simulink model "hopper_6dof_CascadeV2"  (R2025a)
settings: Solver=VariableStepAuto  StartTime=0.0  StopTime=20  RelTol=1e-3
values from neighbouring files (symbols this model uses):
  dcg_dMfu_table = [-0.00694531817472 -0.00694178681649 -0.00693828089331 -0.00693480026996 -0.00693134481199 -0.00692791438575 -0.00692450885835 -0.00692112809769 -0.00691777197246 -0.00691444035208 -0.00691113310675 -0.00690785010743 ... (10000 elements, 100x100)]    [cg_I_LUT.mat]    (also in cg_moi_table_generation.m = zeros(length(ox_masses), length(fu_masses)))
  dcg_dMox_table = [-0.00694531817472 0.00355111679481 0.00356856249576 0.00358595402521 0.00360329160721 0.00362057546465 0.00363780581927 0.00365498289166 0.0036721069013 0.00368917806651 0.00370619660452 0.00372316273141 ... (10000 elements, 100x100)]    [cg_I_LUT.mat]    (also in cg_moi_table_generation.m = zeros(length(ox_masses), length(fu_masses)))
  dI_dMfu_table = [0.00582660125 0.00582660125 0.00582660125 0.00582660125 0.00582660125 0.00582660125 0.00582660125 0.00582660125 0.00582660125 0.00582660125 0.00582660125 0.00582660125 ... (90000 elements, 100x100x9)]    [cg_I_LUT.mat]    (also in cg_moi_table_generation.m = zeros(length(ox_masses), length(fu_masses), 9))
  dI_dMox_table = [0.00582660125 0.00582660125 0.00582660125 0.00582660125 0.00582660125 0.00582660125 0.00582660125 0.00582660125 0.00582660125 0.00582660125 0.00582660125 0.00582660125 ... (90000 elements, 100x100x9)]    [cg_I_LUT.mat]    (also in cg_moi_table_generation.m = zeros(length(ox_masses), length(fu_masses), 9))
  engine_cg = IN.engine_cg    [cg_moi_table_generation.m]    (also in cg_moi_test.m = 0.3556)
  fu_masses = [0 0.131313131313 0.262626262626 0.393939393939 0.525252525253 0.656565656566 0.787878787879 0.919191919192 1.05050505051 1.18181818182 1.31313131313 1.44444444444 ... (100 elements, 1x100)]    [cg_I_LUT.mat]    (also in cg_moi_table_generation.m = linspace(0,IN.propulsion.fuel_mass,100))
  ox_masses = [0 0.161616161616 0.323232323232 0.484848484848 0.646464646465 0.808080808081 0.969696969697 1.13131313131 1.29292929293 1.45454545455 1.61616161616 1.77777777778 ... (100 elements, 1x100)]    [cg_I_LUT.mat]    (also in cg_moi_table_generation.m = linspace(0,IN.propulsion.oxidizer_mass,100))
undefined symbols (not defined in the file or in its folder): bp, cg_init, IN, MoI_init, OUT, r_leg_1, r_leg_2, r_leg_3, r_leg_4, TANKS, tbl1, tbl2
libraries: matrix_library x18, slpidlib x13, dspindex x2, aerolibanim x1, SignalEditorBlockLib x1, aerolibutil x1
(part 1 of 3)
settings Model: Creator=asing  LastModifiedBy=Espin
settings DebuggingCC: SignalInfNanChecking=warning

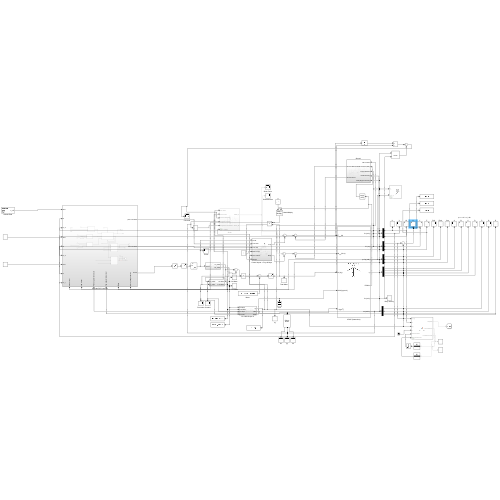
[thumbnail: Simulink's stored preview of the top-level diagram]
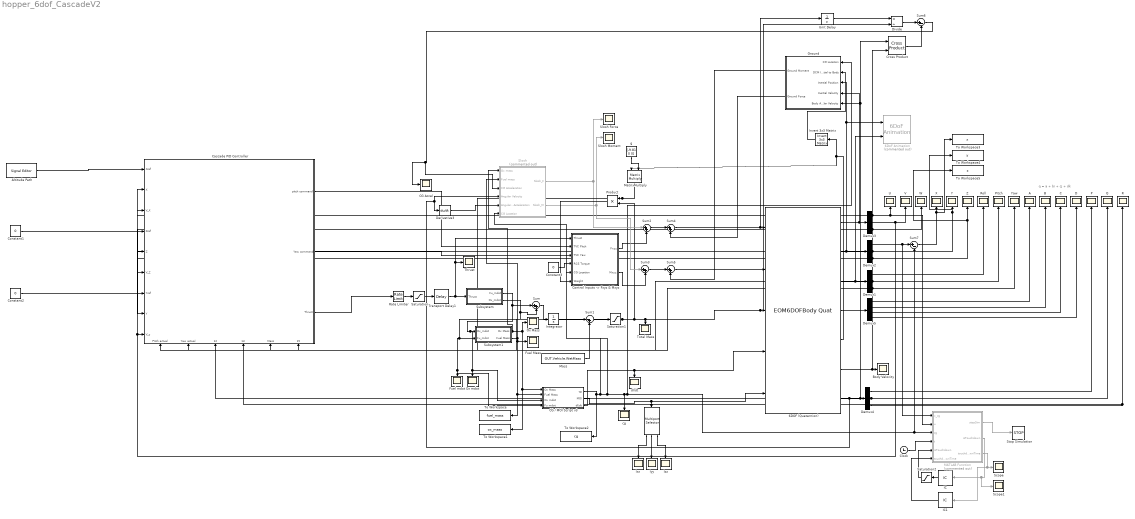
== system hopper_6dof_CascadeV2 ==
  note: q = a + bi + cj + dk
  " " : dspindex/Multiport Selector  rowsOrCols=Rows  idxCellArray={1,2,3}  idxErrMode=Clip Index
      settings: LibrarySourceBlock=|
      | dsphdlsupportsigmgmt/Multiport
      | Selector
  6DOF (Quaternion) : EOM6DOFBodyQuat  mtype=Custom Variable  xme_0=[cg_init 0 0]
  6DoF Animation : aerolibanim/6DoF Animation  Commented=on  u1=[0 4000 -2000 2000 -5000 -3000]  u2=0.1  u3=1.0  u4=[4000 0 -5000]  u5=Fly alongside  u6=[2000 500 -3150]  u7=10  u8=on
  A : Scope
      settings: ActiveDisplayYMinimum=0.99999999995691624  ActiveDisplayYMaximum=1.0000000000047871  DataLoggingVariableName=ScopeData12
  Altitude Path : SignalEditorBlockLib/Signal Editor  FileName=trajectory2.mat  ActiveScenario=scenario  ActiveSignal=z_ref  IsBus=off  OutputBusObjectStr=Bus: BusObject  SampleTime=0  ZeroCross=off  OutputAfterFinalValue=Setting to zero  Unit=inherit  PreserveSignalName=on  ApplySigPropsToAllScenarios=on  ApplySigPropsToAllSignals=off  SignalPropertySource=Dialog parameters
  B : Scope
      settings: ActiveDisplayYMinimum=-1  ActiveDisplayYMaximum=1  DataLoggingVariableName=ScopeData13
  Body Velocity : Scope
      settings: ActiveDisplayYMinimum=-2.8946574443603503  ActiveDisplayYMaximum=19.391983148189578  DataLoggingVariableName=ScopeData29
  C : Scope
      settings: DataLoggingVariableName=ScopeData14
  CG / MOI Script v3 : Subsystem
  CG Accel : Scope
      settings: ActiveDisplayYMinimum=-11.150910258610358  ActiveDisplayYMaximum=2.247247756596932  DataLoggingVariableName=ScopeData33
  Cascade PID Controller : Subsystem
      settings: PortSchema="{\"entries\":[{\"content\":{\"sides\":[{\"content\":{\"connectorIds\":[\"In1\",\"In2\",\"In3\",\"In4\",\"In5\",\"In6\",\"In7\",\"In8\",\"In9\"]},\"type\":\"ConnectorPlacement.EquallySpacedRectSide\",\"uuid\":\"c783e0c4-78fc-4a76-b0b3-9a0d7ec37fa3\"},{\"content\":{\"connectorIds\":[\"Out1\",\"Out2\",\"Out3\"],\"side\":\"RIGHT\"},\"type\":\"ConnectorPlacement.EquallySpacedRectSide\",\"uuid\":\"c1fbc6cd-e8e0-44a7-b5c2-c47c52a42ebb\"},{\"content\":{\"side\":\"TOP\"},\"type\":\"ConnectorPlacement.EquallySpacedRectSide\",\"uuid\":\"09ce9669-ca2f-4231-9dc2-e7ff305f4669\"},{\"content\":{\"connectorIds\":[\"In10\",\"In11\",\"In12\",\"In13\",\"In14\",\"In15\"],\"side\":\"BOTTOM\"},\"type\":\"ConnectorPlacement.EquallySpacedRectSide\",\"uuid\":\"414a52fd-de97-45d1-8e92-1dab180b62e1\"}]},\"type\":\"ConnectorPlacement.EquallySpacedConnector\",\"uuid\":\"cfeff8df-d4aa-41cc-804b-2026e1f59ecf\"}],\"packageUris\":[\"http://schema.mathworks.com/mf0/Connector/R2020b\"],\"version\":\"1.0\"}"
  Clock : Clock
  Constant1 : Constant  Value=0
  Constant2 : Constant  Value=0
  Constant3 : Constant  Value=0
  "Control Inputs -> Fxyz & Mxyz" : Subsystem
  Cross Product : matrix_library/Cross Product
  D : Scope
      settings: DataLoggingVariableName=ScopeData15
  Demux{1..4} (4 alike) : Demux  Outputs=3
  Demux5 : Demux
  Derivative3 : Derivative  CoefficientInTFapproximation=3
  Divide : Product  Inputs=*/
  Fuel Mass : Scope
      settings: ActiveDisplayYMinimum=-1  ActiveDisplayYMaximum=1  DataLoggingVariableName=ScopeData18
  Fuel mdot : Scope
      settings: DataLoggingVariableName=ScopeData20
  "Ground " : Subsystem
  IC : InitialCondition  Value=0
  IC1 : InitialCondition  Value=0
  Integrator : Integrator
  Invert 3x3 Matrix : aerolibutil/Invert  3x3 Matrix
  Ixx : Scope
      settings: ActiveDisplayYMinimum=-0.12644047609192863  ActiveDisplayYMaximum=1.1379642848273579  DataLoggingVariableName=ScopeData21
  Iyy : Scope
      settings: ActiveDisplayYMinimum=-1  ActiveDisplayYMaximum=1  DataLoggingVariableName=ScopeData26
  Izz : Scope
      settings: ActiveDisplayYMinimum=-5.2001669347022288  ActiveDisplayYMaximum=46.801502412320069  DataLoggingVariableName=ScopeData27
  MATLAB Function : MATLAB Function  Commented=on  TreatAsAtomicUnit=on
  Mass : Constant  Value=OUT.Vehicle.WetMass
  MatrixMultiply : Product  Multiplication=Matrix(*)
  Ox Mass : Scope
      settings: ActiveDisplayYMinimum=-1  ActiveDisplayYMaximum=1  DataLoggingVariableName=ScopeData17
  Ox mdot : Scope
      settings: ActiveDisplayYMinimum=-1  ActiveDisplayYMaximum=1  DataLoggingVariableName=ScopeData19
  P : Scope
      settings: ActiveDisplayYMinimum=-1  ActiveDisplayYMaximum=1  DataLoggingVariableName=ScopeData9
  Pitch : Scope
      settings: ActiveDisplayYMinimum=-0.27527761186972155  ActiveDisplayYMaximum=0.20077796412190005  DataLoggingVariableName=ScopeData4
  Product : Product
  Q : Scope
      settings: ActiveDisplayYMinimum=-1  ActiveDisplayYMaximum=1  DataLoggingVariableName=ScopeData10
  R : Scope
      settings: ActiveDisplayYMinimum=-1  ActiveDisplayYMaximum=1  DataLoggingVariableName=ScopeData11
  Rate Limiter : RateLimiter  RisingSlewLimit=IN.throttle_valve.rate_limit  FallingSlewLimit=-IN.throttle_valve.rate_limit  SampleTimeMode=inherited
  Roll : Scope
      settings: ActiveDisplayYMinimum=-3.8311926038814774  ActiveDisplayYMaximum=3.879867078950717  DataLoggingVariableName=ScopeData3
  Saturation : Saturate  UpperLimit=IN.propulsion.nominal_thrust * IN.propulsion.throttle_range(2)  LowerLimit=IN.propulsion.nominal_thrust * IN.propulsion.throttle_range(1)
  Saturation1 : Saturate  UpperLimit=OUT.Vehicle.WetMass  LowerLimit=OUT.Vehicle.DryMass
  Saturation2 : Saturate  UpperLimit=1  LowerLimit=0
  Scope : Scope
      settings: ActiveDisplayYMinimum=-0.36773849090650063  ActiveDisplayYMaximum=3.3096464181585059  DataLoggingVariableName=ScopeData47
  Scope1 : Scope
      settings: ActiveDisplayYMinimum=-4.3477372735072848  ActiveDisplayYMaximum=98.44556029431709  DataLoggingVariableName=ScopeData48
  Slosh : Subsystem  Commented=on
  Slosh Force : Scope
      settings: ActiveDisplayYMinimum=-2049.8081863311008  ActiveDisplayYMaximum=855.4571669030571  DataLoggingVariableName=ScopeData32
  Slosh Moment : Scope
      settings: ActiveDisplayYMinimum=-100.37229864380086  ActiveDisplayYMaximum=480.93099551449279  DataLoggingVariableName=ScopeData35
  Stop Simulation : Stop
  Subsystem : Subsystem
  Subsystem1 : Subsystem
  Sum{,2..5} (5 alike) : Sum  Inputs=|++
  Sum1 : Sum  Inputs=|-+
  Sum6 : Sum  Inputs=|+-
  Sum7 : Sum  Inputs=|+-
  Thrust : Scope
      settings: ActiveDisplayYMinimum=-2.2737842613896349E-6  ActiveDisplayYMaximum=1.0528893262676848E-6  DataLoggingVariableName=ScopeData25
  To Workspace : ToWorkspace  VariableName=fuel_mass  SaveFormat=Timeseries  SampleTime=-1
  To Workspace1 : ToWorkspace  VariableName=ox_mass  SaveFormat=Timeseries  SampleTime=-1
  To Workspace2 : ToWorkspace  VariableName=cg  SaveFormat=Timeseries  SampleTime=-1
  To Workspace3 : ToWorkspace  VariableName=x  SaveFormat=Timeseries  SampleTime=-1
  To Workspace4 : ToWorkspace  VariableName=y  SaveFormat=Timeseries  SampleTime=-1
  To Workspace5 : ToWorkspace  VariableName=z  SaveFormat=Timeseries  SampleTime=-1
  Total Mass : Scope
      settings: ActiveDisplayYMinimum=108.3025441390815  ActiveDisplayYMaximum=114.36006324090583  DataLoggingVariableName=ScopeData16
  Transport Delay1 : TransportDelay  DelayTime=IN.throttle_valve_latency
  U : Scope
      settings: ActiveDisplayYMinimum=-4.7998225296675594  ActiveDisplayYMaximum=42.8778253174209  DataLoggingVariableName=ScopeData6
  Unit Delay : UnitDelay  SampleTime=-1  HasFrameUpgradeWarning=on
  V : Scope
      settings: ActiveDisplayYMinimum=-1  ActiveDisplayYMaximum=1  DataLoggingVariableName=ScopeData7
  W : Scope
      settings: ActiveDisplayYMinimum=-1  ActiveDisplayYMaximum=1  DataLoggingVariableName=ScopeData8
  X : Scope
      settings: ActiveDisplayYMinimum=-478.18693686234167  ActiveDisplayYMaximum=1130.6863299978559
  Y : Scope
      settings: ActiveDisplayYMinimum=-1  ActiveDisplayYMaximum=1
  Yaw : Scope
      settings: ActiveDisplayYMinimum=-3.8972561837654429  ActiveDisplayYMaximum=3.8933218717422249  DataLoggingVariableName=ScopeData5
  Z : Scope
      settings: ActiveDisplayYMinimum=-1  ActiveDisplayYMaximum=1  DataLoggingVariableName=ScopeData2
  cg : Scope
      settings: ActiveDisplayYMinimum=1.3271270693254955  ActiveDisplayYMaximum=1.3302680600816481  DataLoggingVariableName=ScopeData23
  dI/dt : Scope
      settings: ActiveDisplayYMinimum=-0.0817382851157486  ActiveDisplayYMaximum=0.00908203167952762  DataLoggingVariableName=ScopeData22
  g : Constant  Value=[-9.81 0 0]
  wires:
  6DOF (Quaternion)/2 -> "Ground "/3(Inertial Position), 6DoF Animation/1, Demux2/1
  6DOF (Quaternion)/3 -> 6DoF Animation/2, Demux1/1
  Demux2/1 -> Sum7/1, MATLAB Function/1(x_cg)
  Demux2/2 -> To Workspace4/1, Y/1, Cascade PID Controller/8(Y)
  Demux2/3 -> Z/1, To Workspace5/1, Cascade PID Controller/5(Z)
  Demux1/1 -> Roll/1
  Demux1/2 -> Pitch/1, Cascade PID Controller/10(Pitch actual)
  Demux1/3 -> Yaw/1, Cascade PID Controller/11(Yaw actual)
  6DOF (Quaternion)/1 -> Demux3/1, "Ground "/4(Inertial Velocity)
  Demux3/1 -> MATLAB Function/2(u), U/1, Cascade PID Controller/3(V_X)
  Demux3/2 -> Cascade PID Controller/2(X), Cascade PID Controller/9(V_y), V/1
  6DOF (Quaternion)/4 -> Demux5/1
  Demux4/1 -> P/1
  Demux4/2 -> Q/1, Cascade PID Controller/12(Pitch angular rate actual)
  Demux4/3 -> Cascade PID Controller/13(Yaw angular rate actual), R/1
  Demux5/1 -> A/1
  Demux5/2 -> B/1
  Demux5/3 -> C/1
  Demux5/4 -> D/1
  Demux3/3 -> W/1, Cascade PID Controller/6(V_Z)
  Subsystem/1(Fu_mdot) -> CG / MOI Script v3/3(Ox mdot), Ox mdot/1, Subsystem1/1(Ox_mdot), Sum/1
  Subsystem/2(Ox_mdot) -> CG / MOI Script v3/4(Fu mdot), Fuel mdot/1, Subsystem1/2(Fu_mdot), Sum/2
  Sum/1 -> Integrator/1
  Integrator/1 -> Sum1/1
  Mass/1 -> Sum1/2
  Sum1/1 -> Saturation1/1
  Saturation1/1 -> Divide/2, 6DOF (Quaternion)/3, Total Mass/1, Product/2, Cascade PID Controller/14(Mass)
  Subsystem1/2(Fuel Mass) -> Fuel Mass/1, CG / MOI Script v3/2(Fuel Mass), To Workspace/1, Slosh/2(Fuel mass)
  CG / MOI Script v3/2(MOI) -> 6DOF (Quaternion)/5, " "/1
  CG / MOI Script v3/3(dI/dt) -> dI/dt/1, 6DOF (Quaternion)/4
  CG / MOI Script v3/1(cg) -> To Workspace2/1, Slosh/6(CG Location), "Ground "/1(CG Location), MATLAB Function/3(cg), Sum7/2, cg/1, "Control Inputs -> Fxyz & Mxyz"/5(CG Location)
  Rate Limiter/1 -> Saturation/1
  Saturation/1 -> Transport Delay1/1
  Cascade PID Controller/3(Thrust) -> Rate Limiter/1
  Cascade PID Controller/1(pitch command) -> "Control Inputs -> Fxyz & Mxyz"/2(TVC Pitch)
  Cascade PID Controller/2(Yaw command) -> "Control Inputs -> Fxyz & Mxyz"/3(TVC Yaw)
  Constant3/1 -> "Control Inputs -> Fxyz & Mxyz"/4(RCS Torque)
  " "/1 -> Ixx/1
  " "/2 -> Iyy/1
  " "/3 -> Izz/1
  g/1 -> MatrixMultiply/2
  6DOF (Quaternion)/5 -> MatrixMultiply/1, Invert 3x3 Matrix/1
  "Control Inputs -> Fxyz & Mxyz"/1(Fxyz) -> Sum2/2
  Slosh/1(Slosh_F) -> Sum2/1, Slosh Force/1
  "Control Inputs -> Fxyz & Mxyz"/2(Mxyz) -> Sum3/2
  Derivative3/1 -> Slosh/5(Angular Acceleration)
  Subsystem1/1(Ox Mass) -> Slosh/1(Ox mass), CG / MOI Script v3/1(Ox Mass), To Workspace1/1, Ox Mass/1
  6DOF (Quaternion)/6 -> Cross Product/2, Body Velocity/1
  6DOF (Quaternion)/7 -> "Ground "/5(Body Angular Velocity), Cross Product/1, Demux4/1, Derivative3/1, Slosh/4(Angular Velocity)
  Slosh/2(Slosh_M) -> Sum3/1, Slosh Moment/1
  Transport Delay1/1 -> Subsystem/1(Thrust), Thrust/1, "Control Inputs -> Fxyz & Mxyz"/1("Thrust ")
  MatrixMultiply/1 -> Cascade PID Controller/15(Gravity Compensation), Product/1
  Product/1 -> "Control Inputs -> Fxyz & Mxyz"/6(Weight)
  Invert 3x3 Matrix/1 -> "Ground "/2(DCM Inertial to Body)
  Sum2/1 -> Sum4/1
  Sum3/1 -> Sum5/1
  Sum5/1 -> 6DOF (Quaternion)/2
  Sum4/1 -> Unit Delay/1, 6DOF (Quaternion)/1
  "Ground "/1(Ground Moment) -> Sum5/2
  Cross Product/1 -> Sum6/2
  Divide/1 -> Sum6/1
  Sum6/1 -> Slosh/3(CG Acceleration), CG Accel/1
  Unit Delay/1 -> Divide/1
  MATLAB Function/1(stopSim) -> Stop Simulation/1
  Clock/1 -> MATLAB Function/4(t)
  MATLAB Function/2(isTouchdown) -> Scope1/1, IC/1
  IC/1 -> Saturation2/1
  MATLAB Function/3(touchdownTime) -> IC1/1, Scope/1
  IC1/1 -> MATLAB Function/6("touchdownTime ")
  "Ground "/2(Ground Force) -> Sum4/2
  Saturation2/1 -> MATLAB Function/5("isTouchdown ")
  Sum7/1 -> To Workspace3/1, X/1
  Altitude Path/1 -> Cascade PID Controller/1(Xref)
  Constant1/1 -> Cascade PID Controller/4(Zref)
  Constant2/1 -> Cascade PID Controller/7(Yref)

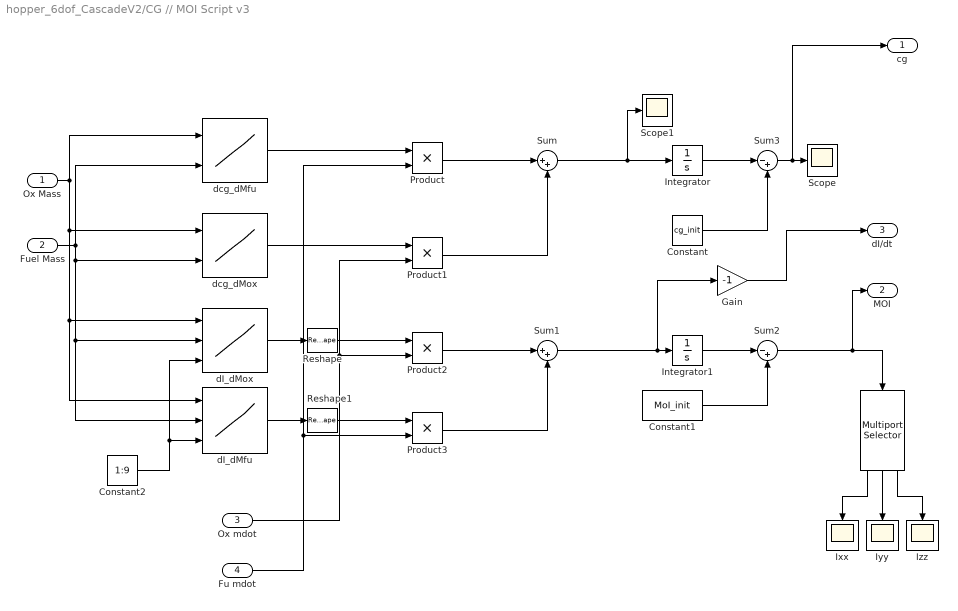
== system hopper_6dof_CascadeV2/CG // MOI Script v3 ==
  Ox Mass : Inport
  Fuel Mass : Inport  Port=2
  Ox mdot : Inport  Port=3
  Fu mdot : Inport  Port=4
  " " : dspindex/Multiport Selector  rowsOrCols=Rows  idxCellArray={1,2,3}  idxErrMode=Clip Index
      settings: LibrarySourceBlock=|
      | dsphdlsupportsigmgmt/Multiport
      | Selector
  Constant : Constant  Value=cg_init
  Constant1 : Constant  Value=MoI_init
  Constant2 : Constant  Value=1:9
  Gain : Gain  Gain=-1
  Integrator : Integrator
  Integrator1 : Integrator
  Ixx : Scope
      settings: ActiveDisplayYMinimum=-0.12644047609192863  ActiveDisplayYMaximum=1.1379642848273579  DataLoggingVariableName=ScopeData19
  Iyy : Scope
      settings: ActiveDisplayYMinimum=30.163212884427733  ActiveDisplayYMaximum=49.780093450314517  DataLoggingVariableName=ScopeData20
  Izz : Scope
      settings: ActiveDisplayYMinimum=-2.8210574648941242  ActiveDisplayYMaximum=25.389517184047122  DataLoggingVariableName=ScopeData22
  Product{,1..3} (4 alike) : Product
  Reshape : Reshape  OutputDimensionality=Customize  OutputDimensions=[3,3]
  Reshape1 : Reshape  OutputDimensionality=Customize  OutputDimensions=[3,3]
  Scope : Scope
      settings: ActiveDisplayYMinimum=-1  ActiveDisplayYMaximum=1  DataLoggingVariableName=ScopeData18
  Scope1 : Scope
      settings: ActiveDisplayYMinimum=-4.6566294760866378E-5  ActiveDisplayYMaximum=0.00041926302445695129  DataLoggingVariableName=ScopeData41
  Sum : Sum  Inputs=|++
  Sum1 : Sum  Inputs=|++
  Sum2 : Sum  Inputs=|-+
  Sum3 : Sum  Inputs=|-+
  dI_dMfu : Lookup_n-D  NumberOfTableDimensions=3  BreakpointsForDimension1=ox_masses  BreakpointsForDimension2=fu_masses  BreakpointsForDimension3=1:9  Table=dI_dMfu_table  InternalRulePriority=Speed  RndMeth=Simplest
      settings: InputPortMap=u0,u1,u2
  dI_dMox : Lookup_n-D  NumberOfTableDimensions=3  BreakpointsForDimension1=ox_masses  BreakpointsForDimension2=fu_masses  BreakpointsForDimension3=1:9  Table=dI_dMox_table  InternalRulePriority=Speed  RndMeth=Simplest
      settings: InputPortMap=u0,u1,u2
  dcg_dMfu : Lookup_n-D  BreakpointsForDimension1=ox_masses  BreakpointsForDimension2=fu_masses  BreakpointsForDimension3=[5, 7]  Table=dcg_dMfu_table  InternalRulePriority=Speed  RndMeth=Simplest
      settings: InputPortMap=u0,u1
  dcg_dMox : Lookup_n-D  BreakpointsForDimension1=ox_masses  BreakpointsForDimension2=fu_masses  BreakpointsForDimension3=[5, 7]  Table=dcg_dMox_table  InternalRulePriority=Speed  RndMeth=Simplest
      settings: InputPortMap=u0,u1
  cg : Outport
  MOI : Outport  Port=2
  dI/dt : Outport  Port=3
  wires:
  Ox Mass/1 -> dI_dMfu/1, dI_dMox/1, dcg_dMox/1, dcg_dMfu/1
  Fuel Mass/1 -> dI_dMfu/2, dI_dMox/2, dcg_dMox/2, dcg_dMfu/2
  dcg_dMfu/1 -> Product/1
  Ox mdot/1 -> Product2/2, Product1/2
  dcg_dMox/1 -> Product1/1
  Fu mdot/1 -> Product3/2, Product/2
  dI_dMox/1 -> Reshape/1
  dI_dMfu/1 -> Reshape1/1
  Product/1 -> Sum/1
  Product1/1 -> Sum/2
  Product2/1 -> Sum1/1
  Product3/1 -> Sum1/2
  Sum/1 -> Scope1/1, Integrator/1
  Integrator/1 -> Sum3/1
  Constant/1 -> Sum3/2
  Sum3/1 -> cg/1, Scope/1
  Sum1/1 -> Gain/1, Integrator1/1
  Integrator1/1 -> Sum2/1
  Constant1/1 -> Sum2/2
  Reshape/1 -> Product2/1
  Reshape1/1 -> Product3/1
  Constant2/1 -> dI_dMfu/3, dI_dMox/3
  " "/2 -> Iyy/1
  " "/1 -> Ixx/1
  " "/3 -> Izz/1
  Sum2/1 -> MOI/1, " "/1
  Gain/1 -> dI/dt/1

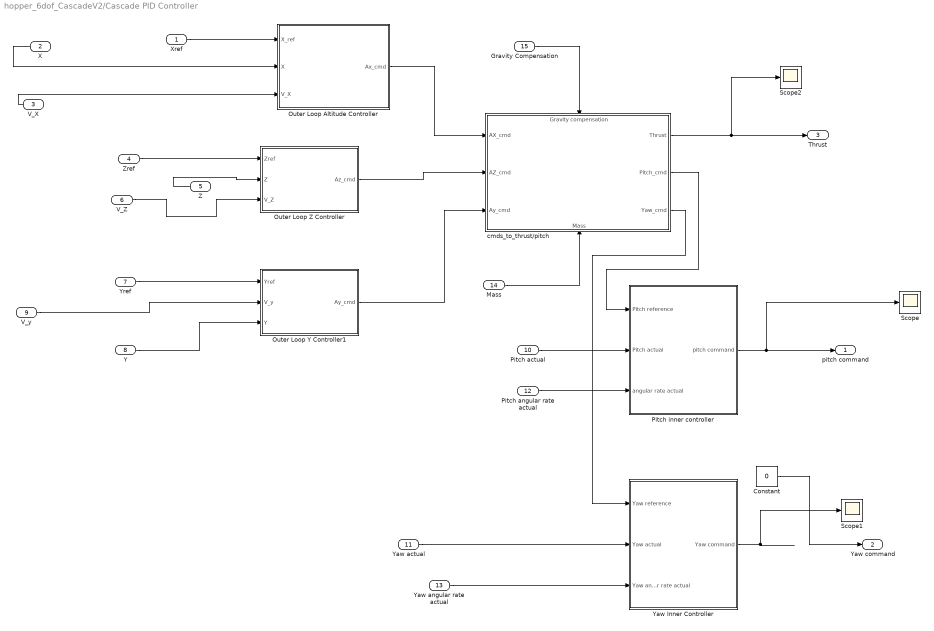
== system hopper_6dof_CascadeV2/Cascade PID Controller ==
  Xref : Inport
  X : Inport  Port=2
  V_X : Inport  Port=3
  Zref : Inport  Port=4
  Z : Inport  Port=5
  V_Z : Inport  Port=6
  Yref : Inport  Port=7
  Y : Inport  Port=8
  V_y : Inport  Port=9
  Pitch actual : Inport  Port=10
  Yaw actual : Inport  Port=11
  Pitch angular rate actual : Inport  Port=12
  Yaw angular rate actual : Inport  Port=13
  Mass : Inport  Port=14
  Gravity Compensation : Inport  Port=15
  Constant : Constant  Value=0
  Outer Loop Altitude Controller : Subsystem
  Outer Loop Y Controller1 : Subsystem
  Outer Loop Z Controller : Subsystem
  Pitch inner controller : Subsystem
  Scope : Scope
      settings: ActiveDisplayYMinimum=-1  ActiveDisplayYMaximum=1  DataLoggingVariableName=ScopeData49
  Scope1 : Scope
      settings: ActiveDisplayYMinimum=-0.44971008329322881  ActiveDisplayYMaximum=0.49286047045357118  DataLoggingVariableName=ScopeData50
  Scope2 : Scope
      settings: ActiveDisplayYMinimum=-1  ActiveDisplayYMaximum=1  DataLoggingVariableName=ScopeData51
  Yaw Inner Controller : Subsystem
  cmds_to_thrust/pitch : Subsystem
      settings: PortSchema="{\"entries\":[{\"content\":{\"sides\":[{\"content\":{\"connectorIds\":[\"In1\",\"In2\",\"In3\"]},\"type\":\"ConnectorPlacement.EquallySpacedRectSide\",\"uuid\":\"64e97352-3d4c-4be0-aecf-a9288b6b77be\"},{\"content\":{\"connectorIds\":[\"Out1\",\"Out2\",\"Out3\"],\"side\":\"RIGHT\"},\"type\":\"ConnectorPlacement.EquallySpacedRectSide\",\"uuid\":\"af625be9-6f04-400a-90a0-f34b6d0a4442\"},{\"content\":{\"connectorIds\":[\"In4\"],\"side\":\"TOP\"},\"type\":\"ConnectorPlacement.EquallySpacedRectSide\",\"uuid\":\"00313782-667a-4601-ba9c-abadbcaead95\"},{\"content\":{\"connectorIds\":[\"In5\"],\"side\":\"BOTTOM\"},\"type\":\"ConnectorPlacement.EquallySpacedRectSide\",\"uuid\":\"a503756a-d495-4001-a372-b56d80b9a67c\"}]},\"type\":\"ConnectorPlacement.EquallySpacedConnector\",\"uuid\":\"2e03bf61-6dd9-4fa2-9389-4888adc8c832\"}],\"packageUris\":[\"http://schema.mathworks.com/mf0/Connector/R2020b\"],\"version\":\"1.0\"}"
  pitch command : Outport
  Yaw command : Outport  Port=2
  Thrust : Outport  Port=3
  wires:
  Yaw angular rate actual/1 -> Yaw Inner Controller/3(Yaw angular rate actual)
  Zref/1 -> Outer Loop Z Controller/1(Zref)
  V_X/1 -> Outer Loop Altitude Controller/3(V_X)
  cmds_to_thrust/pitch/3(Yaw_cmd) -> Yaw Inner Controller/1(Yaw reference)
  Outer Loop Altitude Controller/1(Ax_cmd) -> cmds_to_thrust/pitch/1(AX_cmd)
  Outer Loop Y Controller1/1(Ay_cmd) -> cmds_to_thrust/pitch/3(Ay_cmd)
  Outer Loop Z Controller/1(Az_cmd) -> cmds_to_thrust/pitch/2(AZ_cmd)
  cmds_to_thrust/pitch/2(Pitch_cmd) -> Pitch inner controller/1(Pitch reference)
  Mass/1 -> cmds_to_thrust/pitch/5(Mass)
  V_y/1 -> Outer Loop Y Controller1/2(V_y)
  Y/1 -> Outer Loop Y Controller1/3(Y)
  Yaw Inner Controller/1(Yaw command) -> Scope1/1
  V_Z/1 -> Outer Loop Z Controller/3(V_Z)
  Xref/1 -> Outer Loop Altitude Controller/1(X_ref)
  Pitch inner controller/1(pitch command) -> pitch command/1, Scope/1
  X/1 -> Outer Loop Altitude Controller/2(X)
  Pitch angular rate actual/1 -> Pitch inner controller/3(angular rate actual)
  Yaw actual/1 -> Yaw Inner Controller/2(Yaw actual)
  Pitch actual/1 -> Pitch inner controller/2(Pitch actual)
  Z/1 -> Outer Loop Z Controller/2(Z)
  Yref/1 -> Outer Loop Y Controller1/1(Yref)
  Gravity Compensation/1 -> cmds_to_thrust/pitch/4(Gravity compensation)
  cmds_to_thrust/pitch/1(Thrust) -> Thrust/1, Scope2/1
  Constant/1 -> Yaw command/1

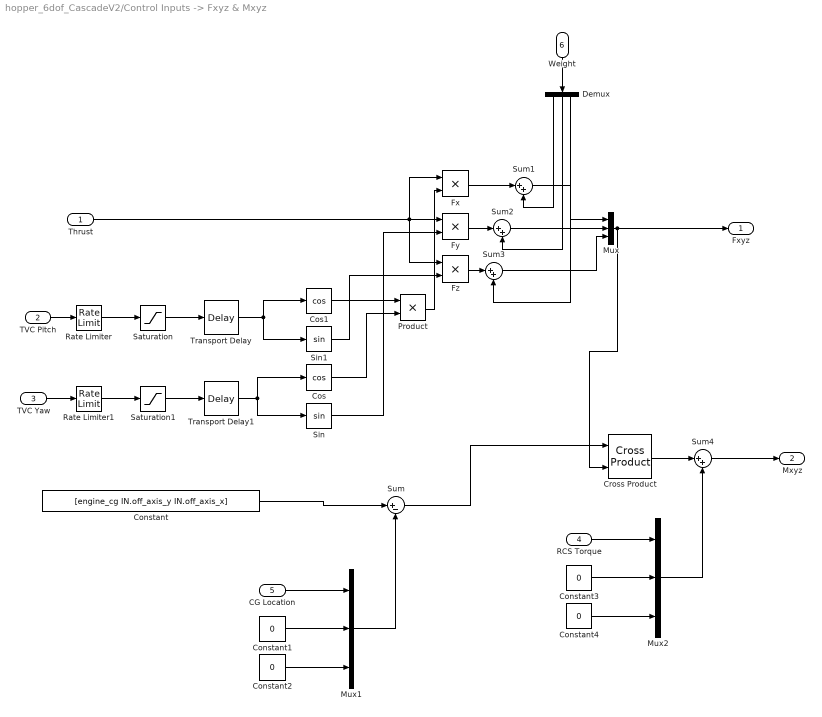
== system hopper_6dof_CascadeV2/Control Inputs -> Fxyz & Mxyz ==
  "Thrust " : Inport
  TVC Pitch : Inport  Port=2
  TVC Yaw : Inport  Port=3
  RCS Torque : Inport  Port=4
  CG Location : Inport  Port=5
  Weight : Inport  Port=6
  Constant : Constant  Value=[engine_cg IN.off_axis_y IN.off_axis_x]
  Constant{1..4} (4 alike) : Constant  Value=0
  Cos : Trigonometry  Operator=cos
  Cos1 : Trigonometry  Operator=cos
  Cross Product : matrix_library/Cross Product
  Demux : Demux  Outputs=3
  Fx : Product
  Fy : Product
  Fz : Product
  Mux : Mux  Inputs=3
  Mux1 : Mux  Inputs=3
  Mux2 : Mux  Inputs=3
  Product : Product
  Rate Limiter : RateLimiter  RisingSlewLimit=IN.tvc.max_gimbal_rate  FallingSlewLimit=-IN.tvc.max_gimbal_rate  SampleTimeMode=inherited
  Rate Limiter1 : RateLimiter  RisingSlewLimit=IN.tvc.max_gimbal_rate  FallingSlewLimit=-IN.tvc.max_gimbal_rate  SampleTimeMode=inherited
  Saturation : Saturate  UpperLimit=IN.tvc.max_gimbal_angle  LowerLimit=-IN.tvc.max_gimbal_angle
  Saturation1 : Saturate  UpperLimit=IN.tvc.max_gimbal_angle  LowerLimit=-IN.tvc.max_gimbal_angle  LinearizeAsGain=off
  Sin : Trigonometry
  Sin1 : Trigonometry
  Sum : Sum  Inputs=|+-
  Sum{1..4} (4 alike) : Sum  Inputs=|++
  Transport Delay : TransportDelay  DelayTime=IN.tvc.actuator_latency
  Transport Delay1 : TransportDelay  DelayTime=IN.tvc.actuator_latency
  Fxyz : Outport
  Mxyz : Outport  Port=2
  wires:
  TVC Yaw/1 -> Rate Limiter1/1
  TVC Pitch/1 -> Rate Limiter/1
  Cos1/1 -> Product/1
  Cos/1 -> Product/2
  Product/1 -> Fx/2
  "Thrust "/1 -> Fx/1, Fy/1, Fz/1
  Sin/1 -> Fy/2
  Sin1/1 -> Fz/2
  Mux/1 -> Cross Product/2, Fxyz/1
  Sum3/1 -> Mux/3
  Fx/1 -> Sum1/1
  Sum1/1 -> Mux/1
  Weight/1 -> Demux/1
  Demux/1 -> Sum1/2
  Fy/1 -> Sum2/1
  Sum2/1 -> Mux/2
  Fz/1 -> Sum3/1
  Demux/2 -> Sum2/2
  Demux/3 -> Sum3/2
  Constant/1 -> Sum/1
  CG Location/1 -> Mux1/1
  Constant1/1 -> Mux1/2
  Constant2/1 -> Mux1/3
  Mux1/1 -> Sum/2
  Sum/1 -> Cross Product/1
  Cross Product/1 -> Sum4/1
  Sum4/1 -> Mxyz/1
  RCS Torque/1 -> Mux2/1
  Constant3/1 -> Mux2/2
  Mux2/1 -> Sum4/2
  Constant4/1 -> Mux2/3
  Saturation/1 -> Transport Delay/1
  Rate Limiter/1 -> Saturation/1
  Rate Limiter1/1 -> Saturation1/1
  Saturation1/1 -> Transport Delay1/1
  Transport Delay/1 -> Sin1/1, Cos1/1
  Transport Delay1/1 -> Sin/1, Cos/1

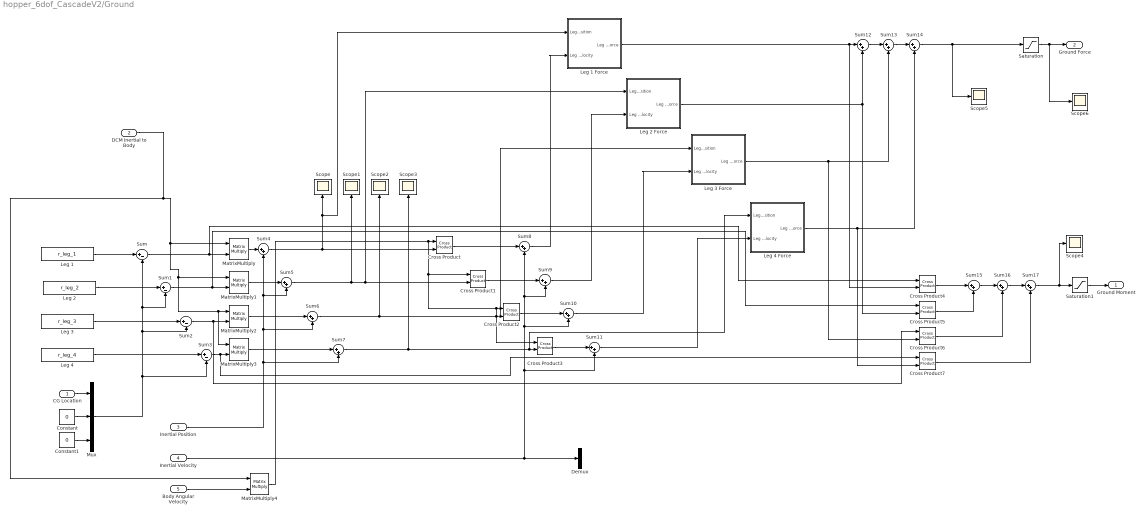
== system hopper_6dof_CascadeV2/Ground  ==
  CG Location : Inport
  DCM Inertial to Body : Inport  Port=2
  Inertial Position : Inport  Port=3
  Inertial Velocity : Inport  Port=4
  Body Angular Velocity : Inport  Port=5
  Constant : Constant  Value=0
  Constant1 : Constant  Value=0
  Cross Product{,1..7} (8 alike) : matrix_library/Cross Product
  Demux : Demux  Outputs=3
  Leg 1 : Constant  Value=r_leg_1
  Leg 1 Force : Subsystem
  Leg 2 : Constant  Value=r_leg_2
  Leg 2 Force : Subsystem
  Leg 3 : Constant  Value=r_leg_3
  Leg 3 Force : Subsystem
  Leg 4 : Constant  Value=r_leg_4
  Leg 4 Force : Subsystem
  MatrixMultiply{,1..4} (5 alike) : Product  Multiplication=Matrix(*)
  Mux : Mux  Inputs=3
  Saturation : Saturate  UpperLimit=inf  LowerLimit=0
  Saturation1 : Saturate  UpperLimit=inf  LowerLimit=0
  Scope{,1..6} (7 alike) : Scope
      Scope settings: ActiveDisplayYMinimum=-19.811154048207108  ActiveDisplayYMaximum=167.31101950999761  DataLoggingVariableName=ScopeData24
      Scope1 settings: ActiveDisplayYMinimum=182.10765195211306  ActiveDisplayYMaximum=183.93696889205802  DataLoggingVariableName=ScopeData30
      Scope2 settings: DataLoggingVariableName=ScopeData31
      Scope3 settings: DataLoggingVariableName=ScopeData42
      Scope4 settings: ActiveDisplayYMinimum=-335392.54571492958  ActiveDisplayYMaximum=333330.77297425125  DataLoggingVariableName=ScopeData43
      Scope5 settings: ActiveDisplayYMinimum=-102144.15432406096  ActiveDisplayYMaximum=890940.43760258122  DataLoggingVariableName=ScopeData44
      Scope6 settings: ActiveDisplayYMinimum=-98409.281906018819  ActiveDisplayYMaximum=885683.53715416964  DataLoggingVariableName=ScopeData45
  Sum{,1..3} (4 alike) : Sum  Inputs=|+-
  Sum{4..17} (14 alike) : Sum  Inputs=|++
  Ground Moment : Outport
  Ground Force : Outport  Port=2
  wires:
  CG Location/1 -> Mux/1
  Constant/1 -> Mux/2
  Constant1/1 -> Mux/3
  Leg 1/1 -> Sum/1
  Leg 2/1 -> Sum1/1
  Leg 3/1 -> Sum2/1
  Leg 4/1 -> Sum3/1
  Mux/1 -> Sum3/2, Sum1/2, Sum/2, Sum2/2
  Sum/1 -> Cross Product4/1, MatrixMultiply/2
  DCM Inertial to Body/1 -> MatrixMultiply4/1, MatrixMultiply1/1, MatrixMultiply3/1, MatrixMultiply2/1, MatrixMultiply/1
  Sum1/1 -> Cross Product5/1, MatrixMultiply1/2
  Sum2/1 -> Cross Product6/1, MatrixMultiply2/2
  Sum3/1 -> Cross Product7/1, MatrixMultiply3/2
  MatrixMultiply3/1 -> Sum7/1
  MatrixMultiply2/1 -> Sum6/1
  MatrixMultiply1/1 -> Sum5/1
  MatrixMultiply/1 -> Sum4/1
  Inertial Position/1 -> Sum7/2, Sum6/2, Sum5/2, Sum4/2
  Sum4/1 -> Scope/1, Leg 1 Force/1(Leg Position), Cross Product/2
  Sum5/1 -> Cross Product1/2, Leg 2 Force/1(Leg Position), Scope1/1
  Sum6/1 -> Leg 3 Force/1(Leg Position), Cross Product2/2, Scope2/1
  Sum7/1 -> Leg 4 Force/1(Leg Position), Cross Product3/2, Scope3/1
  Body Angular Velocity/1 -> MatrixMultiply4/2
  MatrixMultiply4/1 -> Cross Product1/1, Cross Product3/1, Cross Product2/1, Cross Product/1
  Cross Product/1 -> Sum8/1
  Cross Product1/1 -> Sum9/1
  Cross Product2/1 -> Sum10/1
  Cross Product3/1 -> Sum11/1
  Inertial Velocity/1 -> Demux/1, Sum11/2, Sum10/2, Sum9/2, Sum8/2
  Leg 1 Force/1(Leg 1 Force) -> Cross Product4/2, Sum12/1
  Leg 2 Force/1(Leg 2 Force) -> Cross Product5/2, Sum12/2
  Sum12/1 -> Sum13/1
  Leg 3 Force/1(Leg 3 Force) -> Cross Product6/2, Sum13/2
  Sum13/1 -> Sum14/1
  Leg 4 Force/1(Leg 4 Force) -> Cross Product7/2, Sum14/2
  Sum14/1 -> Saturation/1, Scope5/1
  Cross Product4/1 -> Sum15/1
  Sum15/1 -> Sum16/1
  Cross Product5/1 -> Sum15/2
  Cross Product6/1 -> Sum16/2
  Sum16/1 -> Sum17/1
  Cross Product7/1 -> Sum17/2
  Sum17/1 -> Scope4/1, Saturation1/1
  Sum8/1 -> Leg 1 Force/2(Leg Velocity)
  Sum9/1 -> Leg 2 Force/2(Leg Velocity)
  Sum10/1 -> Leg 3 Force/2(Leg Velocity)
  Sum11/1 -> Leg 4 Force/2(Leg Velocity)
  Saturation/1 -> Ground Force/1, Scope6/1
  Saturation1/1 -> Ground Moment/1

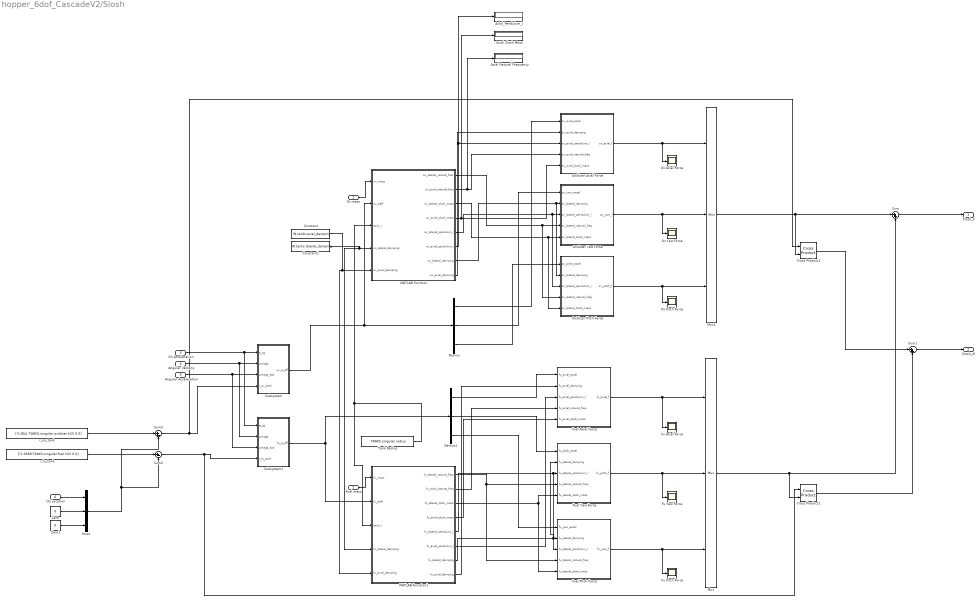
== system hopper_6dof_CascadeV2/Slosh ==
  Ox mass : Inport
  Fuel mass : Inport  Port=2
  CG Acceleration : Inport  Port=3
  Angular Velocity : Inport  Port=4
  Angular Acceleration : Inport  Port=5
  CG Location : Inport  Port=6
  Axial Natural Frequency : Display
  Axial Slosh Mass : Display
  Axial_Pendulum_l : Display
  Constant : Constant  Value=IN.tanks.axial_damping
  Constant1 : Constant  Value=IN.tanks.lateral_damping
  Cross Product1 : matrix_library/Cross Product
  Cross Product2 : matrix_library/Cross Product
  Demux : Demux  Outputs=3
  Demux1 : Demux  Outputs=3
  Fu Axial Force : Scope
      settings: ActiveDisplayYMinimum=-43.769852074588144  ActiveDisplayYMaximum=34.138533481497277  DataLoggingVariableName=ScopeData38
  Fu Pitch Force : Scope
      settings: ActiveDisplayYMinimum=-202.25487847173252  ActiveDisplayYMaximum=208.52247446010225  DataLoggingVariableName=ScopeData40
  Fu Yaw Force : Scope
      settings: ActiveDisplayYMinimum=-203.787600574714  ActiveDisplayYMaximum=201.11273706154645  DataLoggingVariableName=ScopeData39
  Fuel Axial Force : Subsystem
  Fuel Pitch Force : Subsystem
  Fuel Yaw Force : Subsystem
  MATLAB Function : MATLAB Function  TreatAsAtomicUnit=on
  MATLAB Function1 : MATLAB Function  TreatAsAtomicUnit=on
  Mux : Mux  Inputs=3
  Mux1 : Mux  Inputs=3
  Mux2 : Mux  Inputs=3
  Ox Axial Force : Scope
      settings: ActiveDisplayYMinimum=-1177.5392999006397  ActiveDisplayYMaximum=580.93477401137238  DataLoggingVariableName=ScopeData34
  Ox Pitch Force : Scope
      settings: ActiveDisplayYMinimum=-226684.22745760108  ActiveDisplayYMaximum=112402.51217436095  DataLoggingVariableName=ScopeData36
  Ox Yaw Force : Scope
      settings: ActiveDisplayYMinimum=-39.505095525762954  ActiveDisplayYMaximum=64.191645366542915  DataLoggingVariableName=ScopeData37
  Oxidizer Axial Force : Subsystem
  Oxidizer Pitch Force : Subsystem
  Oxidizer Yaw Force : Subsystem
  Subsystem : Subsystem
  Subsystem1 : Subsystem
  Sum : Sum  Inputs=|++
  Sum1 : Sum  Inputs=|++
  Sum2 : Sum  Inputs=|+-
  Sum3 : Sum  Inputs=|+-
  Tank Radius : Constant  Value=TANKS.singular.radius  SampleTime=-1
  Zero : Constant  Value=0  OutDataTypeStr=Inherit: Inherit via back propagation
  Zero1 : Constant  Value=0  OutDataTypeStr=Inherit: Inherit via back propagation
  r_fu_tank : Constant  Value=[(1.0668-TANKS.singular.fuel.h/2) 0 0]
  r_ox_tank : Constant  Value=[(1.854 -TANKS.singular.oxidizer.h/2) 0 0]
  Slosh_F : Outport
  Slosh_M : Outport  Port=2
  wires:
  Ox mass/1 -> MATLAB Function/1(ox_mass)
  CG Acceleration/1 -> Subsystem/1(a_cg), Subsystem1/1(a_cg)
  Angular Velocity/1 -> Subsystem/2(omega), Subsystem1/2(omega)
  Angular Acceleration/1 -> Subsystem/3(omega_dot), Subsystem1/3(omega_dot)
  Fuel mass/1 -> MATLAB Function1/1(fu_mass)
  Subsystem/1(ox_a_eff) -> Demux/1, MATLAB Function/2(ox_aeff)
  Subsystem1/1(fu_a_eff) -> Demux1/1, MATLAB Function1/2(fu_aeff)
  Demux/1 -> Oxidizer Axial Force/1(ox_axial_accel)
  Demux/2 -> Oxidizer Yaw Force/1(ox_yaw_accel)
  Demux/3 -> Oxidizer Pitch Force/1(ox_pitch_accel)
  Demux1/1 -> Fuel Axial Force/1(fu_axial_accel)
  Demux1/2 -> Fuel Yaw Force/1(fu_pitch_accel)
  Demux1/3 -> Fuel Pitch Force/1(fu_yaw_accel)
  MATLAB Function/1(ox_lateral_natural_freq) -> Oxidizer Yaw Force/4(ox_lateral_natural_freq), Oxidizer Pitch Force/4(ox_lateral_natural_freq)
  MATLAB Function/2(ox_axial_natural_freq) -> Axial Natural Frequency/1, Oxidizer Axial Force/4(ox_axial_natural_freq)
  MATLAB Function/3(ox_lateral_slosh_mass) -> Oxidizer Yaw Force/5(ox_lateral_slosh_mass), Oxidizer Pitch Force/5(ox_lateral_slosh_mass)
  MATLAB Function/4(ox_axial_slosh_mass) -> Axial Slosh Mass/1, Oxidizer Axial Force/5(ox_axial_slosh_mass)
  MATLAB Function/5(ox_lateral_pendulum_l) -> Oxidizer Yaw Force/3(ox_lateral_pendulum_l), Oxidizer Pitch Force/3(ox_lateral_pendulum_l)
  MATLAB Function/6(ox_axial_pendulum_l) -> Axial_Pendulum_l/1, Oxidizer Axial Force/3(ox_axial_pendulum_l)
  MATLAB Function/7(ox_lateral_damping) -> Oxidizer Pitch Force/2(ox_lateral_damping), Oxidizer Yaw Force/2(ox_lateral_damping)
  MATLAB Function/8(ox_axial_damping) -> Oxidizer Axial Force/2(ox_axial_damping)
  MATLAB Function1/1(fu_lateral_natural_freq) -> Fuel Yaw Force/4(fu_lateral_natural_freq), Fuel Pitch Force/4(fu_lateral_natural_freq)
  MATLAB Function1/2(fu_axial_natural_freq) -> Fuel Axial Force/4(fu_axial_natural_freq)
  MATLAB Function1/3(fu_lateral_slosh_mass) -> Fuel Pitch Force/5(fu_lateral_slosh_mass), Fuel Yaw Force/5(fu_lateral_slosh_mass)
  MATLAB Function1/4(fu_axial_slosh_mass) -> Fuel Axial Force/5(fu_axial_slosh_mass)
  MATLAB Function1/5(fu_lateral_pendulum_l) -> Fuel Pitch Force/3(fu_lateral_pendulum_l), Fuel Yaw Force/3(fu_lateral_pendulum_l)
  MATLAB Function1/6(fu_axial_pendulum_l) -> Fuel Axial Force/3(fu_axial_pendulum_l)
  MATLAB Function1/7(fu_lateral_damping) -> Fuel Yaw Force/2(fu_lateral_damping), Fuel Pitch Force/2(fu_lateral_damping)
  MATLAB Function1/8(fu_axial_damping) -> Fuel Axial Force/2(fu_axial_damping)
  Fuel Axial Force/1(fu_axial_f) -> Fu Axial Force/1, Mux/1
  Fuel Yaw Force/1(fu_pitch_f) -> Fu Yaw Force/1, Mux/2
  Fuel Pitch Force/1(fu_yaw_f) -> Fu Pitch Force/1, Mux/3
  Oxidizer Axial Force/1(ox_axial_f) -> Ox Axial Force/1, Mux1/1
  Oxidizer Yaw Force/1(ox_yaw_f) -> Ox Yaw Force/1, Mux1/2
  Oxidizer Pitch Force/1(ox_pitch_f) -> Ox Pitch Force/1, Mux1/3
  Mux1/1 -> Cross Product1/2, Sum/1
  Mux/1 -> Sum/2, Cross Product2/2
  Sum/1 -> Slosh_F/1
  Cross Product1/1 -> Sum1/1
  Cross Product2/1 -> Sum1/2
  Sum1/1 -> Slosh_M/1
  Tank Radius/1 -> MATLAB Function1/3(tank_r), MATLAB Function/3(tank_r)
  CG Location/1 -> Mux2/1
  Zero/1 -> Mux2/2
  Zero1/1 -> Mux2/3
  r_ox_tank/1 -> Sum3/1
  r_fu_tank/1 -> Sum2/1
  Mux2/1 -> Sum2/2, Sum3/2
  Sum3/1 -> Cross Product1/1, Subsystem/4(r_ox_tank)
  Sum2/1 -> Cross Product2/1, Subsystem1/4(r_fu_tank)
  Constant/1 -> MATLAB Function/5("ox_axial_damping "), MATLAB Function1/5("fu_axial_damping ")
  Constant1/1 -> MATLAB Function/4("ox_lateral_damping "), MATLAB Function1/4("fu_lateral_damping ")

== system hopper_6dof_CascadeV2/Subsystem ==
  Thrust : Inport
  Fuel mdot : Lookup_n-D  NumberOfTableDimensions=1  BreakpointsForDimension1=bp  Table=tbl2  InternalRulePriority=Speed  RndMeth=Simplest
  Ox mdot : Lookup_n-D  NumberOfTableDimensions=1  BreakpointsForDimension1=bp  Table=tbl1  InternalRulePriority=Speed  RndMeth=Simplest
  Fu_mdot : Outport
  Ox_mdot : Outport  Port=2
  wires:
  Thrust/1 -> Ox mdot/1, Fuel mdot/1
  Fuel mdot/1 -> Fu_mdot/1
  Ox mdot/1 -> Ox_mdot/1

== system hopper_6dof_CascadeV2/Subsystem1 ==
  Ox_mdot : Inport
  Fu_mdot : Inport  Port=2
  Integrator : Integrator
  Integrator1 : Integrator
  Ox Mass1 : Constant  Value=IN.propulsion.oxidizer_mass
  Ox Mass2 : Constant  Value=IN.propulsion.fuel_mass
  Saturation : Saturate  UpperLimit=IN.propulsion.oxidizer_mass  LowerLimit=0
  Saturation1 : Saturate  UpperLimit=IN.propulsion.fuel_mass  LowerLimit=0
  Sum : Sum  Inputs=|-+
  Sum1 : Sum  Inputs=|-+
  Ox Mass : Outport
  Fuel Mass : Outport  Port=2
  wires:
  Ox_mdot/1 -> Integrator/1
  Integrator/1 -> Sum/1
  Ox Mass1/1 -> Sum/2
  Sum/1 -> Saturation/1
  Saturation/1 -> Ox Mass/1
  Sum1/1 -> Saturation1/1
  Saturation1/1 -> Fuel Mass/1
  Fu_mdot/1 -> Integrator1/1
  Ox Mass2/1 -> Sum1/2
  Integrator1/1 -> Sum1/1

== system hopper_6dof_CascadeV2/Cascade PID Controller/Outer Loop Altitude Controller ==
  X_ref : Inport
  X : Inport  Port=2
  V_X : Inport  Port=3
  Abs : Abs  SaturateOnIntegerOverflow=off
  Gain1 : Gain  Gain=1.5
  PID Controller : slpidlib/PID Controller  Controller=PID  Form=Parallel  TimeDomain=Discrete-time  UseExternalTs=off  SampleTime=.02  IntegratorMethod=Forward Euler  FilterMethod=Forward Euler  ControllerParametersSource=internal  P=-10.7939994356276  I=-0.435354080790359  UseKiTs=off  D=-31.9383700868144  UseExternalDerivativeSource=off  N=71.8360137365129  UseFilter=off  TunerSelectOption=Transfer Function Based (PID Tuner App)  InitialConditionSource=internal  InitialConditionForIntegrator=0  InitialConditionForFilter=0  DifferentiatorICPrevScaledInput=0  ExternalReset=none  TrackingMode=off  Kt=1  LimitOutput=off  SatLimitsSource=internal  UpperSaturationLimit=inf  LowerSaturationLimit=-inf  LinearizeAsGain=on  AntiWindupMode=none  Kb=1  LimitIntegrator=off  UpperIntegratorSaturationLimit=inf  LowerIntegratorSaturationLimit=-inf  POutMin=[]  POutMax=[]  IOutMin=[]  IOutMax=[]  DOutMin=[]  DOutMax=[]  NOutMin=[]  NOutMax=[]  SumOutMin=[]  SumOutMax=[]  SaturationOutMin=[]  SaturationOutMax=[]  PParamMin=[]  PParamMax=[]  IParamMin=[]  IParamMax=[]  DParamMin=[]  DParamMax=[]  NParamMin=[]  NParamMax=[]  KbParamMin=[]  KbParamMax=[]  KtParamMin=[]  KtParamMax=[]  KbOutMin=[]  KbOutMax=[]  KtOutMin=[]  KtOutMax=[]  IntegratorOutMin=[]  IntegratorOutMax=[]  FilterOutMin=[]  FilterOutMax=[]  SumI1OutMin=[]  SumI1OutMax=[]  SumI2OutMin=[]  SumI2OutMax=[]  SumI3OutMin=[]  SumI3OutMax=[]  SumI4OutMin=[]  SumI4OutMax=[]  SumDOutMin=[]  SumDOutMax=[]  DifferentiatorOutMin=[]  DifferentiatorOutMax=[]  FilterDiffOutCoefMin=[]  FilterDiffOutCoefMax=[]  ReciprocalOutMin=[]  ReciprocalOutMax=[]  SumDenOutMin=[]  SumDenOutMax=[]  SumNumOutMin=[]  SumNumOutMax=[]  DivideOutMin=[]  DivideOutMax=[]  UdiffTsProdOutMin=[]  UdiffTsProdOutMax=[]  NTsProdOutMin=[]  NTsProdOutMax=[]  UintegralTsProdOutMin=[]  UintegralTsProdOutMax=[]  UngainTsProdOutMin=[]  UngainTsProdOutMax=[]  ClampingZeroOutDataTypeStr=Inherit: Inherit via back propagation  ClampingZeroOutMin=[]  ClampingZeroOutMax=[]  FilterDenConstantOutDataTypeStr=Inherit: Inherit via back propagation  FilterDenConstantOutMin=[]  FilterDenConstantOutMax=[]  PCopyOutDataTypeStr=Inherit: Inherit via back propagation  PCopyOutMin=[]  PCopyOutMax=[]  NCopyOutDataTypeStr=Inherit: Inherit via back propagation  NCopyOutMin=[]  NCopyOutMax=[]  IntegratorContinuousStateAttributes=''  IntegratorStateMustResolveToSignalObject=off  IntegratorRTWStateStorageClass=Auto  FilterContinuousStateAttributes=''  FilterStateMustResolveToSignalObject=off  FilterRTWStateStorageClass=Auto  ParallelPVariant=InternalParameters  IdealPVariant=Disabled  IVariant=InternalParameters  DVariant=InternalParameters  IntegratorVariant=Discrete  SatVariant=Disabled  AWVariant=Passthrough  PCopyVariant=Disabled  TRVariant=Disabled  FdbkBlocksVariant=Forward  IdealPFdbkVariant=Disabled  SatFdbkVariant=Disabled  DerivativeFilterVariant=Differentiator  NVariant=Passthrough  NCopyVariant=Disabled_SignalSpec  FilterICVariant=InternalICsDifferentiator  IntegratorICVariant=InternalICs  ExternalResetVariant=Disabled  TRSumVariant=Passthrough  SumFdbkVariant=Disabled  SumVariant=Sum_PID  TsampFilterVariant=InternalTs  TsampNgainVariant=Passthrough  TsampIntegralVariant=Disabled_SignalSpec  ExternalSaturationOutDataTypeStr=Inherit: Same as second input  DerivativeSourceVariant=ErrorSignal  PreIntVariant=InternalPreInt
  PID Controller1 : slpidlib/PID Controller  Controller=PID  Form=Parallel  TimeDomain=Discrete-time  UseExternalTs=off  SampleTime=.02  IntegratorMethod=Forward Euler  FilterMethod=Forward Euler  ControllerParametersSource=internal  P=10788.2186722466  I=172.428431118727  UseKiTs=off  D=12100.5369383532  UseExternalDerivativeSource=off  N=71.8360137365129  UseFilter=off  TunerSelectOption=Transfer Function Based (PID Tuner App)  InitialConditionSource=internal  InitialConditionForIntegrator=0  InitialConditionForFilter=0  DifferentiatorICPrevScaledInput=0  ExternalReset=none  TrackingMode=off  Kt=1  LimitOutput=off  SatLimitsSource=internal  UpperSaturationLimit=inf  LowerSaturationLimit=-inf  LinearizeAsGain=on  AntiWindupMode=none  Kb=1  LimitIntegrator=off  UpperIntegratorSaturationLimit=inf  LowerIntegratorSaturationLimit=-inf  POutMin=[]  POutMax=[]  IOutMin=[]  IOutMax=[]  DOutMin=[]  DOutMax=[]  NOutMin=[]  NOutMax=[]  SumOutMin=[]  SumOutMax=[]  SaturationOutMin=[]  SaturationOutMax=[]  PParamMin=[]  PParamMax=[]  IParamMin=[]  IParamMax=[]  DParamMin=[]  DParamMax=[]  NParamMin=[]  NParamMax=[]  KbParamMin=[]  KbParamMax=[]  KtParamMin=[]  KtParamMax=[]  KbOutMin=[]  KbOutMax=[]  KtOutMin=[]  KtOutMax=[]  IntegratorOutMin=[]  IntegratorOutMax=[]  FilterOutMin=[]  FilterOutMax=[]  SumI1OutMin=[]  SumI1OutMax=[]  SumI2OutMin=[]  SumI2OutMax=[]  SumI3OutMin=[]  SumI3OutMax=[]  SumI4OutMin=[]  SumI4OutMax=[]  SumDOutMin=[]  SumDOutMax=[]  DifferentiatorOutMin=[]  DifferentiatorOutMax=[]  FilterDiffOutCoefMin=[]  FilterDiffOutCoefMax=[]  ReciprocalOutMin=[]  ReciprocalOutMax=[]  SumDenOutMin=[]  SumDenOutMax=[]  SumNumOutMin=[]  SumNumOutMax=[]  DivideOutMin=[]  DivideOutMax=[]  UdiffTsProdOutMin=[]  UdiffTsProdOutMax=[]  NTsProdOutMin=[]  NTsProdOutMax=[]  UintegralTsProdOutMin=[]  UintegralTsProdOutMax=[]  UngainTsProdOutMin=[]  UngainTsProdOutMax=[]  ClampingZeroOutDataTypeStr=Inherit: Inherit via back propagation  ClampingZeroOutMin=[]  ClampingZeroOutMax=[]  FilterDenConstantOutDataTypeStr=Inherit: Inherit via back propagation  FilterDenConstantOutMin=[]  FilterDenConstantOutMax=[]  PCopyOutDataTypeStr=Inherit: Inherit via back propagation  PCopyOutMin=[]  PCopyOutMax=[]  NCopyOutDataTypeStr=Inherit: Inherit via back propagation  NCopyOutMin=[]  NCopyOutMax=[]  IntegratorContinuousStateAttributes=''  IntegratorStateMustResolveToSignalObject=off  IntegratorRTWStateStorageClass=Auto  FilterContinuousStateAttributes=''  FilterStateMustResolveToSignalObject=off  FilterRTWStateStorageClass=Auto  ParallelPVariant=InternalParameters  IdealPVariant=Disabled  IVariant=InternalParameters  DVariant=InternalParameters  IntegratorVariant=Discrete  SatVariant=Disabled  AWVariant=Passthrough  PCopyVariant=Disabled  TRVariant=Disabled  FdbkBlocksVariant=Forward  IdealPFdbkVariant=Disabled  SatFdbkVariant=Disabled  DerivativeFilterVariant=Differentiator  NVariant=Passthrough  NCopyVariant=Disabled_SignalSpec  FilterICVariant=InternalICsDifferentiator  IntegratorICVariant=InternalICs  ExternalResetVariant=Disabled  TRSumVariant=Passthrough  SumFdbkVariant=Disabled  SumVariant=Sum_PID  TsampFilterVariant=InternalTs  TsampNgainVariant=Passthrough  TsampIntegralVariant=Disabled_SignalSpec  ExternalSaturationOutDataTypeStr=Inherit: Same as second input  DerivativeSourceVariant=ErrorSignal  PreIntVariant=InternalPreInt
  Scope : Scope
      settings: ActiveDisplayYMinimum=-6.471697230538922  ActiveDisplayYMaximum=34.872052769461078  DataLoggingVariableName=ScopeData27
  Scope2 : Scope
      settings: ActiveDisplayYMinimum=-1450.1308335174933  ActiveDisplayYMaximum=480.08268664272219  DataLoggingVariableName=ScopeData29
  Scope3 : Scope
      settings: ActiveDisplayYMinimum=-2628.2294879970932  ActiveDisplayYMaximum=1011.4759807937319  DataLoggingVariableName=ScopeData30
  Sum : Sum  Inputs=|+-
  Sum1 : Sum  Inputs=|+-
  Ax_cmd : Outport
  wires:
  X_ref/1 -> Sum/1
  Sum/1 -> Scope2/1, PID Controller/1
  V_X/1 -> Gain1/1
  Sum1/1 -> Scope/1, PID Controller1/1
  X/1 -> Scope3/1, Sum/2
  PID Controller/1 -> Sum1/1
  Gain1/1 -> Sum1/2
  PID Controller1/1 -> Ax_cmd/1
